simulink model "Gen_Battery_Model_02"  (R2017a)
settings: Solver=VariableStepAuto  StartTime=0.0  StopTime=3600  RelTol=1e-3
settings Model: Creator=hlope  LastModifiedBy=hlope
settings DataIOCC: ExternalInput=[t u]  LoadExternalInput=on  ReturnWorkspaceOutputs=on  OutputSaveName=Vt

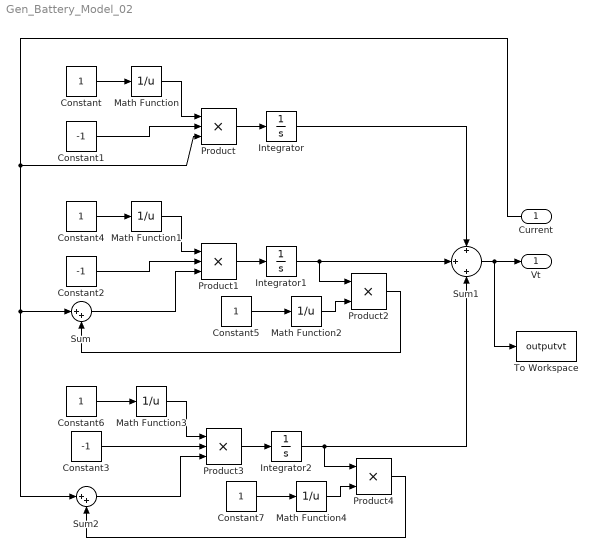
== system Gen_Battery_Model_02 ==
  Current : Inport
  Constant{,4..7} (5 alike) : Constant
  Constant1 : Constant  Value=-1
  Constant2 : Constant  Value=-1
  Constant3 : Constant  Value=-1
  Integrator : Integrator
  Integrator1 : Integrator
  Integrator2 : Integrator
  Math Function{,1..4} (5 alike) : Math  Operator=reciprocal  SaturateOnIntegerOverflow=on
  Product : Product  Inputs=3
  Product1 : Product  Inputs=3
  Product2 : Product
  Product3 : Product  Inputs=3
  Product4 : Product
  Sum : Sum  Inputs=|++
  Sum1 : Sum  Inputs=+|+|+
  Sum2 : Sum  Inputs=|++
  To Workspace : ToWorkspace  VariableName=outputvt  SampleTime=-1
  Vt : Outport
  wires:
  Constant/1 -> Math Function/1
  Math Function/1 -> Product/1
  Product/1 -> Integrator/1
  Constant1/1 -> Product/2
  Constant4/1 -> Math Function1/1
  Math Function1/1 -> Product1/1
  Constant2/1 -> Product1/2
  Product1/1 -> Integrator1/1
  Sum/1 -> Product1/3
  Integrator1/1 -> Product2/1, Sum1/2
  Constant5/1 -> Math Function2/1
  Math Function2/1 -> Product2/2
  Product2/1 -> Sum/2
  Integrator/1 -> Sum1/1
  Integrator2/1 -> Sum1/3, Product4/1
  Sum2/1 -> Product3/3
  Constant7/1 -> Math Function4/1
  Constant3/1 -> Product3/2
  Math Function4/1 -> Product4/2
  Product3/1 -> Integrator2/1
  Math Function3/1 -> Product3/1
  Product4/1 -> Sum2/2
  Constant6/1 -> Math Function3/1
  Sum1/1 -> To Workspace/1, Vt/1
  Current/1 -> Product/3, Sum2/1, Sum/1
